simulink model "H_bot_model"  (R2021b)
settings: Solver=VariableStepAuto  StartTime=0.0  StopTime=1  RelTol=1e-3
values from neighbouring files (symbols this model uses):
  D = zeros(2)    [CoreXY_analysis_func.m]    (also in tuning.m)
  Km = 0.04025    [CoreXY_analysis_func.m]    (also in tuning.m)
undefined symbols (not defined in the file or in its folder): current_limit, D_inv, k_d, k_i, k_p, L_terminal, R_terminal, Z
libraries: cstblocks x2, slpidlib x2, simulink x1
settings Model: Creator=trent  LastModifiedBy=andre

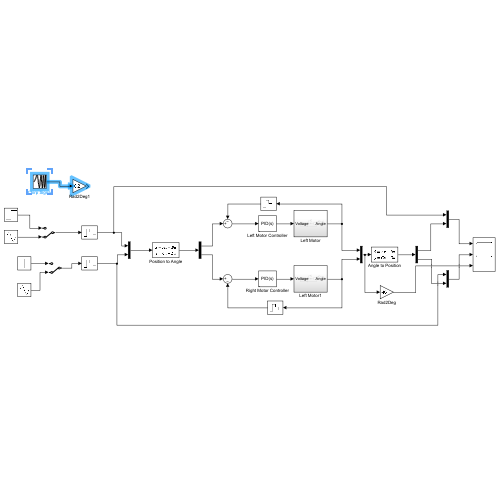
[thumbnail: Simulink's stored preview of the top-level diagram]
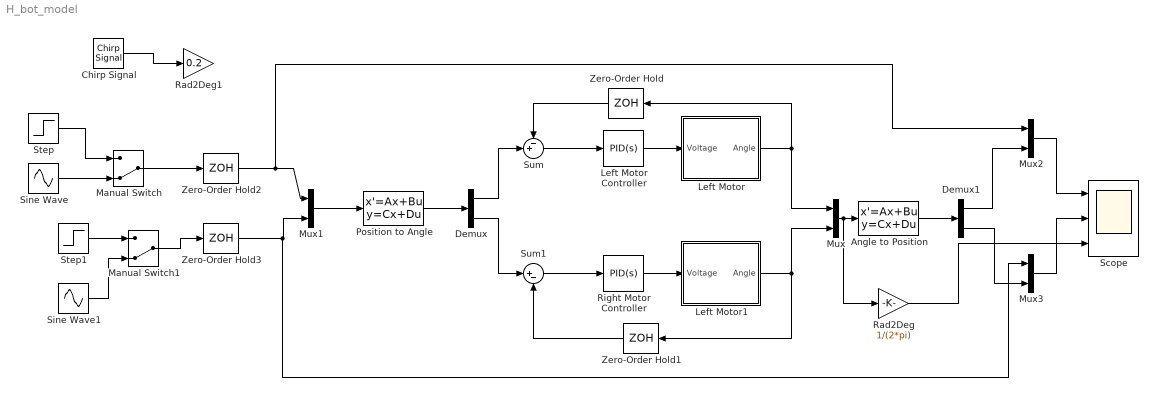
== system H_bot_model ==
  Angle to Position : StateSpace  A=Z  B=Z  C=Z  D=D  InitialCondition=0
  Chirp Signal : simulink/Sources/Chirp Signal  f1=.5  T=10  f2=5
  Demux : Demux  Outputs=2
  Demux1 : Demux  Outputs=2
  Left Motor : Subsystem
  Left Motor Controller : slpidlib/PID Controller  Controller=PID  Form=Parallel  TimeDomain=Continuous-time  UseExternalTs=off  SampleTime=-1  IntegratorMethod=Forward Euler  FilterMethod=Forward Euler  ControllerParametersSource=internal  P=k_p  I=k_i  D=k_d  UseFilter=on  N=2*1000  TunerSelectOption=Transfer Function Based (PID Tuner App)  InitialConditionSource=internal  InitialConditionForIntegrator=0  InitialConditionForFilter=0  DifferentiatorICPrevScaledInput=0  ExternalReset=none  TrackingMode=off  Kt=1  LimitOutput=off  SatLimitsSource=internal  UpperSaturationLimit=inf  LowerSaturationLimit=-inf  LinearizeAsGain=on  AntiWindupMode=none  Kb=1  POutMin=[]  POutMax=[]  IOutMin=[]  IOutMax=[]  DOutMin=[]  DOutMax=[]  NOutMin=[]  NOutMax=[]  SumOutMin=[]  SumOutMax=[]  SaturationOutMin=[]  SaturationOutMax=[]  PParamMin=[]  PParamMax=[]  IParamMin=[]  IParamMax=[]  DParamMin=[]  DParamMax=[]  NParamMin=[]  NParamMax=[]  KbParamMin=[]  KbParamMax=[]  KtParamMin=[]  KtParamMax=[]  KbOutMin=[]  KbOutMax=[]  KtOutMin=[]  KtOutMax=[]  IntegratorOutMin=[]  IntegratorOutMax=[]  FilterOutMin=[]  FilterOutMax=[]  SumI1OutMin=[]  SumI1OutMax=[]  SumI2OutMin=[]  SumI2OutMax=[]  SumI3OutMin=[]  SumI3OutMax=[]  SumI4OutMin=[]  SumI4OutMax=[]  SumDOutMin=[]  SumDOutMax=[]  DifferentiatorOutMin=[]  DifferentiatorOutMax=[]  FilterDiffOutCoefMin=[]  FilterDiffOutCoefMax=[]  ReciprocalOutMin=[]  ReciprocalOutMax=[]  SumDenOutMin=[]  SumDenOutMax=[]  SumNumOutMin=[]  SumNumOutMax=[]  DivideOutMin=[]  DivideOutMax=[]  UdiffTsProdOutMin=[]  UdiffTsProdOutMax=[]  NTsProdOutMin=[]  NTsProdOutMax=[]  UintegralTsProdOutMin=[]  UintegralTsProdOutMax=[]  UngainTsProdOutMin=[]  UngainTsProdOutMax=[]  IntegratorContinuousStateAttributes=''  IntegratorStateMustResolveToSignalObject=off  IntegratorRTWStateStorageClass=Auto  FilterContinuousStateAttributes=''  FilterStateMustResolveToSignalObject=off  FilterRTWStateStorageClass=Auto  ParallelPVariant=InternalParameters  IdealPVariant=Disabled  IVariant=InternalParameters  DVariant=InternalParameters  IntegratorVariant=Continuous  SatVariant=Disabled  AWVariant=Passthrough  PCopyVariant=Disabled  TRVariant=Disabled  FdbkBlocksVariant=Forward  IdealPFdbkVariant=Disabled  SatFdbkVariant=Disabled  DerivativeFilterVariant=ContFilter  NVariant=InternalParameters  NCopyVariant=Disabled  FilterICVariant=InternalICsFilter  IntegratorICVariant=InternalICs  ExternalResetVariant=Disabled  TRSumVariant=Passthrough  SumFdbkVariant=Disabled  SumVariant=Sum_PID  TsampFilterVariant=InternalTs  TsampNgainVariant=Passthrough  TsampIntegralVariant=Passthrough  ExternalSaturationOutDataTypeStr=Inherit: Same as second input
  Left Motor1 : Subsystem
  Manual Switch : ManualSwitch  CurrentSetting=0
  Manual Switch1 : ManualSwitch  CurrentSetting=0
  Mux{,1..3} (4 alike) : Mux  Inputs=2
  Position to Angle : StateSpace  A=Z  B=Z  C=Z  D=D_inv  InitialCondition=0
  Rad2Deg : Gain  Gain=1/(2*pi)
  Rad2Deg1 : Gain  Gain=0.2
  Right Motor Controller : slpidlib/PID Controller  Controller=PID  Form=Parallel  TimeDomain=Continuous-time  UseExternalTs=off  SampleTime=-1  IntegratorMethod=Forward Euler  FilterMethod=Forward Euler  ControllerParametersSource=internal  P=k_p  I=k_i  D=k_d  UseFilter=on  N=2*1000  TunerSelectOption=Transfer Function Based (PID Tuner App)  InitialConditionSource=internal  InitialConditionForIntegrator=0  InitialConditionForFilter=0  DifferentiatorICPrevScaledInput=0  ExternalReset=none  TrackingMode=off  Kt=1  LimitOutput=off  SatLimitsSource=internal  UpperSaturationLimit=inf  LowerSaturationLimit=-inf  LinearizeAsGain=on  AntiWindupMode=none  Kb=1  POutMin=[]  POutMax=[]  IOutMin=[]  IOutMax=[]  DOutMin=[]  DOutMax=[]  NOutMin=[]  NOutMax=[]  SumOutMin=[]  SumOutMax=[]  SaturationOutMin=[]  SaturationOutMax=[]  PParamMin=[]  PParamMax=[]  IParamMin=[]  IParamMax=[]  DParamMin=[]  DParamMax=[]  NParamMin=[]  NParamMax=[]  KbParamMin=[]  KbParamMax=[]  KtParamMin=[]  KtParamMax=[]  KbOutMin=[]  KbOutMax=[]  KtOutMin=[]  KtOutMax=[]  IntegratorOutMin=[]  IntegratorOutMax=[]  FilterOutMin=[]  FilterOutMax=[]  SumI1OutMin=[]  SumI1OutMax=[]  SumI2OutMin=[]  SumI2OutMax=[]  SumI3OutMin=[]  SumI3OutMax=[]  SumI4OutMin=[]  SumI4OutMax=[]  SumDOutMin=[]  SumDOutMax=[]  DifferentiatorOutMin=[]  DifferentiatorOutMax=[]  FilterDiffOutCoefMin=[]  FilterDiffOutCoefMax=[]  ReciprocalOutMin=[]  ReciprocalOutMax=[]  SumDenOutMin=[]  SumDenOutMax=[]  SumNumOutMin=[]  SumNumOutMax=[]  DivideOutMin=[]  DivideOutMax=[]  UdiffTsProdOutMin=[]  UdiffTsProdOutMax=[]  NTsProdOutMin=[]  NTsProdOutMax=[]  UintegralTsProdOutMin=[]  UintegralTsProdOutMax=[]  UngainTsProdOutMin=[]  UngainTsProdOutMax=[]  IntegratorContinuousStateAttributes=''  IntegratorStateMustResolveToSignalObject=off  IntegratorRTWStateStorageClass=Auto  FilterContinuousStateAttributes=''  FilterStateMustResolveToSignalObject=off  FilterRTWStateStorageClass=Auto  ParallelPVariant=InternalParameters  IdealPVariant=Disabled  IVariant=InternalParameters  DVariant=InternalParameters  IntegratorVariant=Continuous  SatVariant=Disabled  AWVariant=Passthrough  PCopyVariant=Disabled  TRVariant=Disabled  FdbkBlocksVariant=Forward  IdealPFdbkVariant=Disabled  SatFdbkVariant=Disabled  DerivativeFilterVariant=ContFilter  NVariant=InternalParameters  NCopyVariant=Disabled  FilterICVariant=InternalICsFilter  IntegratorICVariant=InternalICs  ExternalResetVariant=Disabled  TRSumVariant=Passthrough  SumFdbkVariant=Disabled  SumVariant=Sum_PID  TsampFilterVariant=InternalTs  TsampNgainVariant=Passthrough  TsampIntegralVariant=Passthrough  ExternalSaturationOutDataTypeStr=Inherit: Same as second input
  Scope : Scope  NumInputPorts=3
  Sine Wave : Sin  Amplitude=0.1  Frequency=pi  SampleTime=0
  Sine Wave1 : Sin  Amplitude=0.1  Frequency=2*pi  SampleTime=0
  Step : Step  Time=0  SampleTime=0
  Step1 : Step  Time=0  SampleTime=0
  Sum : Sum  Inputs=-+|
  Sum1 : Sum  Inputs=|+-
  Zero-Order Hold : ZeroOrderHold  SampleTime=0.01
  Zero-Order Hold1 : ZeroOrderHold  SampleTime=0.01
  Zero-Order Hold2 : ZeroOrderHold  SampleTime=0.001
  Zero-Order Hold3 : ZeroOrderHold  SampleTime=0.001
  wires:
  Left Motor/1(Angle) -> Mux/1, Zero-Order Hold/1
  Left Motor1/1(Angle) -> Zero-Order Hold1/1, Mux/2
  Mux/1 -> Rad2Deg/1, Angle to Position/1
  Position to Angle/1 -> Demux/1
  Zero-Order Hold3/1 -> Mux3/1, Mux1/2
  Zero-Order Hold2/1 -> Mux2/1, Mux1/1
  Mux1/1 -> Position to Angle/1
  Left Motor Controller/1 -> Left Motor/1(Voltage)
  Right Motor Controller/1 -> Left Motor1/1(Voltage)
  Demux/1 -> Sum/2
  Sum/1 -> Left Motor Controller/1
  Demux/2 -> Sum1/1
  Sum1/1 -> Right Motor Controller/1
  Zero-Order Hold/1 -> Sum/1
  Zero-Order Hold1/1 -> Sum1/2
  Angle to Position/1 -> Demux1/1
  Demux1/1 -> Mux2/2
  Demux1/2 -> Mux3/2
  Mux2/1 -> Scope/1
  Mux3/1 -> Scope/2
  Step/1 -> Manual Switch/1
  Sine Wave/1 -> Manual Switch/2
  Step1/1 -> Manual Switch1/1
  Rad2Deg/1 -> Scope/3
  Chirp Signal/1 -> Rad2Deg1/1
  Manual Switch/1 -> Zero-Order Hold2/1
  Manual Switch1/1 -> Zero-Order Hold3/1
  Sine Wave1/1 -> Manual Switch1/2

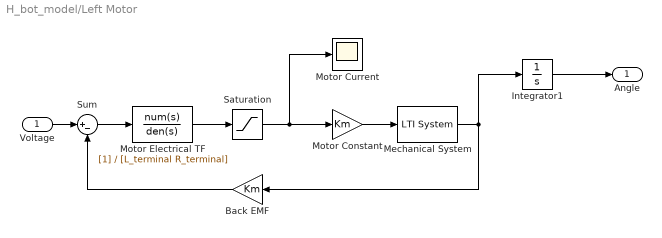
== system H_bot_model/Left Motor ==
  Voltage : Inport
  Back EMF : Gain  Gain=Km
  Integrator1 : Integrator
  Mechanical System : cstblocks/LTI System  sys=Ym  IC=[]
  Motor Constant : Gain  Gain=Km
  Motor Current : Scope
  Motor Electrical TF : TransferFcn  Denominator=[L_terminal R_terminal]
  Saturation : Saturate  UpperLimit=current_limit  LowerLimit=-current_limit
  Sum : Sum  Inputs=|+-
  Angle : Outport
  wires:
  Voltage/1 -> Sum/1
  Sum/1 -> Motor Electrical TF/1
  Motor Constant/1 -> Mechanical System/1
  Mechanical System/1 -> Back EMF/1, Integrator1/1
  Back EMF/1 -> Sum/2
  Integrator1/1 -> Angle/1
  Motor Electrical TF/1 -> Saturation/1
  Saturation/1 -> Motor Current/1, Motor Constant/1

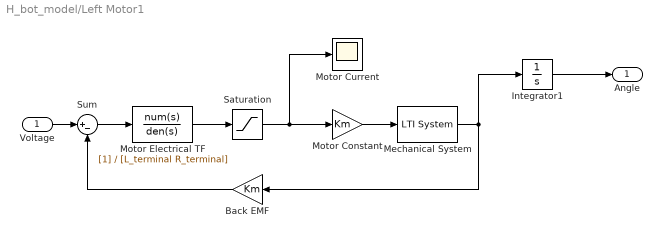
== system H_bot_model/Left Motor1 ==
  Voltage : Inport
  Back EMF : Gain  Gain=Km
  Integrator1 : Integrator
  Mechanical System : cstblocks/LTI System  sys=Ym  IC=[]
  Motor Constant : Gain  Gain=Km
  Motor Current : Scope
  Motor Electrical TF : TransferFcn  Denominator=[L_terminal R_terminal]
  Saturation : Saturate  UpperLimit=current_limit  LowerLimit=-current_limit
  Sum : Sum  Inputs=|+-
  Angle : Outport
  wires:
  Saturation/1 -> Motor Constant/1, Motor Current/1
  Motor Electrical TF/1 -> Saturation/1
  Integrator1/1 -> Angle/1
  Back EMF/1 -> Sum/2
  Mechanical System/1 -> Integrator1/1, Back EMF/1
  Motor Constant/1 -> Mechanical System/1
  Sum/1 -> Motor Electrical TF/1
  Voltage/1 -> Sum/1
